simulink model "Cart_Pendulum_Linear"  (R2019b)
settings: Solver=VariableStepAuto  StartTime=0.0  StopTime=10.0  RelTol=1e-3
undefined symbols (not defined in the file or in its folder): A_mat, B_mat, C_mat, D_mat, K
settings Model: Creator=don  LastModifiedBy=don

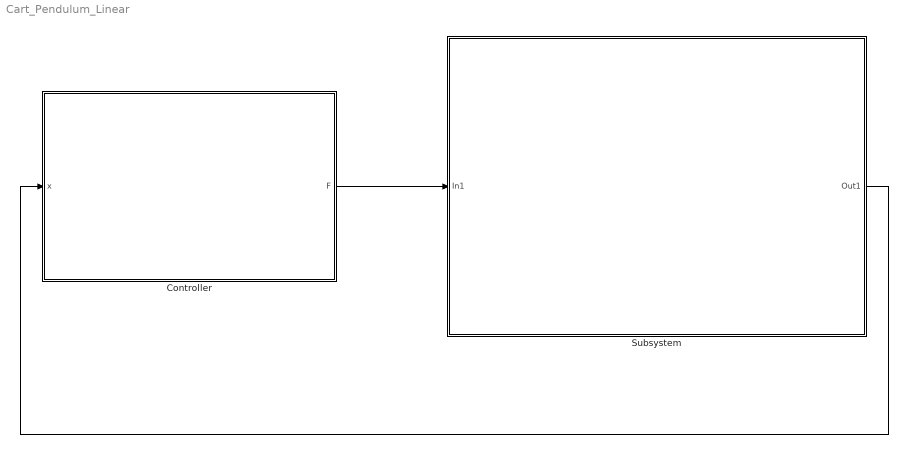
== system Cart_Pendulum_Linear ==
  Controller : Subsystem
  Subsystem : Subsystem
  wires:
  Controller/1(F) -> Subsystem/1(In1)
  Subsystem/1(Out1) -> Controller/1(x)

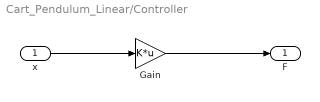
== system Cart_Pendulum_Linear/Controller ==
  x : Inport
  Gain : Gain  Gain=K*u
  F : Outport
  wires:
  x/1 -> Gain/1
  Gain/1 -> F/1

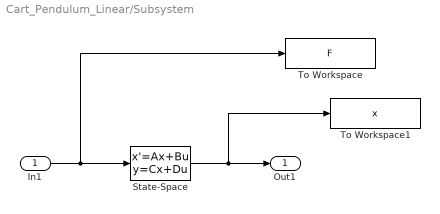
== system Cart_Pendulum_Linear/Subsystem ==
  In1 : Inport
  State-Space : StateSpace  A=A_mat  B=B_mat  C=C_mat  D=D_mat  InitialCondition=0
  To Workspace : ToWorkspace  VariableName=F  SaveFormat=Timeseries  SampleTime=-1
  To Workspace1 : ToWorkspace  VariableName=x  SaveFormat=Timeseries  SampleTime=-1
  Out1 : Outport
  wires:
  In1/1 -> To Workspace/1, State-Space/1
  State-Space/1 -> To Workspace1/1, Out1/1
